simulink model "stpa_brake_manage_maintain"  (R2022a)
settings: Solver=VariableStepAuto  StartTime=0.0  StopTime=10.0  RelTol=1e-3
settings Model: Creator=adije  LastModifiedBy=ayj
settings DebuggingCC: UnconnectedInputMsg=warning  UnconnectedOutputMsg=warning  UnconnectedLineMsg=warning
settings RTWCC: DLArmComputeVersion=19.05

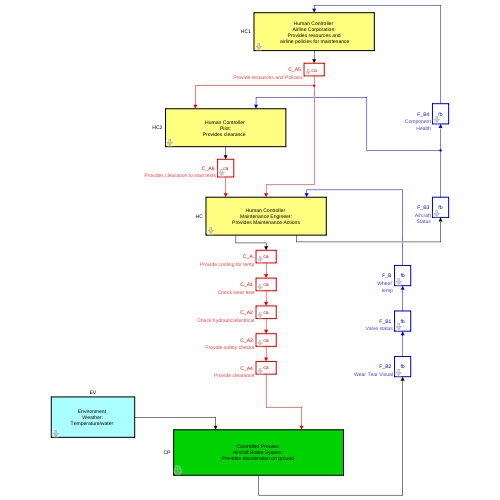
[thumbnail: Simulink's stored preview of the top-level diagram]
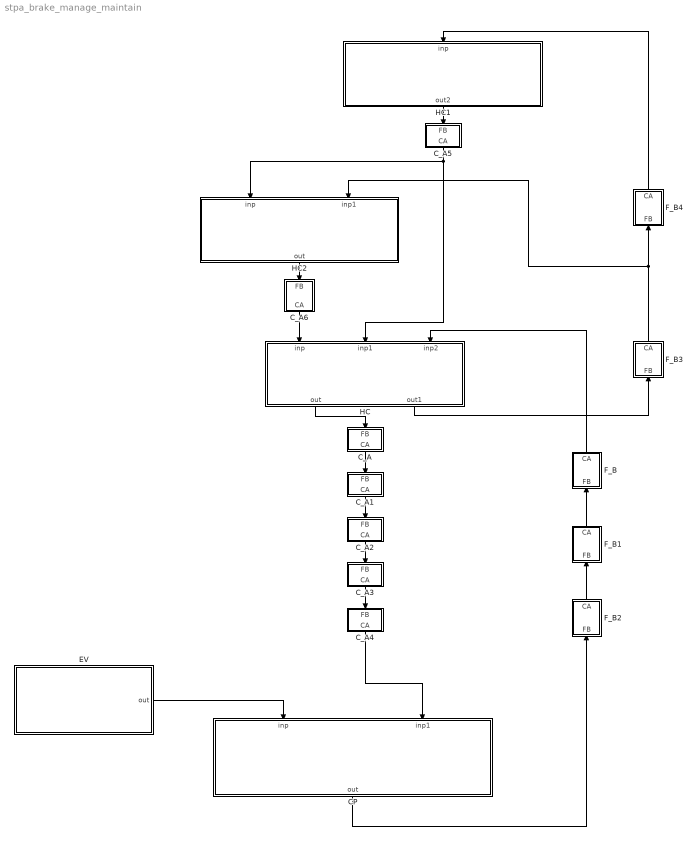
== system stpa_brake_manage_maintain ==
  CP : Subsystem  TreatAsAtomicUnit=on  mask(controlled_process){NAMEFORBLOCK=Aircraft Brake System, DES=Provides deceleration on ground}
      mask prompts: NAMEFORBLOCK "Provide a name for Block"; DES "Provide a description of Responsibility"
      mask help: Say what this controlled process does
      settings: RTWFcnNameOpts=Use subsystem name  RTWFileNameOpts=Use function name
      mask DialogControl Control2 Prompt: ADD Input
      mask DialogControl Control2 Callback:
      | set_param(gcb,'LinkStatus', 'none');
      | h = add_block('simulink/Sources/In1', [gcb '/inp'], 'MakeNameUnique', 'on');
      | hg = add_block('simulink/Sinks/Terminator', [gcb '/term'], 'MakeNameUnique', 'on');
      | hname = get_param(h,'PortHandles');
      | hgname = get_param(hg,'PortHandles');
      | add_line(gcb, hname.Outport(1), hgname.Inport(1));
      mask DialogControl Control3 Prompt: ADD Output
      mask DialogControl Control3 Callback:
      | set_param(gcb,'LinkStatus', 'none');
      | h = add_block('simulink/Sinks/Out1', [gcb '/out'], 'MakeNameUnique', 'on');
      | hg = add_block('simulink/Sources/Ground', [gcb '/gnd'], 'MakeNameUnique', 'on');
      | hname = get_param(h,'PortHandles');
      | hgname = get_param(hg,'PortHandles');
      | add_line(gcb, hgname.Outport(1), hname.Inport(1));
      mask DialogControl Control4 Prompt: REM Input
      mask DialogControl Control4 Callback:
      | set_param(gcb,'LinkStatus', 'none');
      | a=find_system(gcb,'SearchDepth',2,'LookUnderMasks','all','BlockType','Inport');
      | if ~isempty(a)
      | b=get_param(a{1},'PortConnectivity');
      | delete_block(a{1});
      | delete_block(b.DstBlock);
      | delete_line(find_system(gcb, 'SearchDepth',2,'LookUnderMasks','all','FindAll', 'on', 'Type', 'line', 'Connected', 'off'))
      | end
      mask DialogControl Control5 Prompt: REM Output
      mask DialogControl Control5 Callback:
      | set_param(gcb,'LinkStatus', 'none');
      | a=find_system(gcb,'SearchDepth',2,'LookUnderMasks','all','BlockType','Outport');
      | if ~isempty(a)
      | b=get_param(a{1},'PortConnectivity');
      | delete_block(a{1});
      | delete_block(b.SrcBlock);
      | delete_line(find_system(gcb, 'SearchDepth',2,'LookUnderMasks','all','FindAll', 'on', 'Type', 'line', 'Connected', 'off'))
      | end
      mask Display: disp(['Controlled Process \n' NAMEFORBLOCK ':\n' DES])
  C_A : Subsystem  TreatAsAtomicUnit=on  mask(control_action){DES=Provide cooling for temp, UCA1=[#H6] Not providing when temp high, UCA2=[#H6] Providing cooling when not required, UCA3=[#H6] Provide cooling before temprature check, UCA4=[#H6] Provide too long / too short (temp high/low)}
      mask prompts: DES "Provide a description of Control Action"; UCA1 "Not providing causes hazard [link Hazard]"; UCA2 "Providing causes hazard [link Hazard]"; UCA3 "Too early, too late, out of order [link Hazard]"; UCA4 "Stopped too soon, applied too long [link Hazard]"
      mask help:
      | <Source> <Type> <Control Action> <Context> <Link to Hazards>
      | Source = System Above, Type = {provided, not provided ..], Control Action = command
      | from the description, Context = While/When .. Always link to a hazard
      mask init:
      | set_param(gcb,'LinkStatus', 'none');
      settings: AttributesFormatString=%<DES>  RTWFcnNameOpts=Use subsystem name  RTWFileNameOpts=Use function name
      mask Display: disp('ca')
  C_A1 : Subsystem  TreatAsAtomicUnit=on  mask(control_action){DES=Check wear tear, UCA1=[#H7, #H6] Not providing regular checks, UCA2=, UCA3=[#H6] Providing too late, UCA4=[#H7] Takes too long to check}
      mask prompts: DES "Provide a description of Control Action"; UCA1 "Not providing causes hazard [link Hazard]"; UCA2 "Providing causes hazard [link Hazard]"; UCA3 "Too early, too late, out of order [link Hazard]"; UCA4 "Stopped too soon, applied too long [link Hazard]"
      mask help:
      | <Source> <Type> <Control Action> <Context> <Link to Hazards>
      | Source = System Above, Type = {provided, not provided ..], Control Action = command
      | from the description, Context = While/When .. Always link to a hazard
      mask init:
      | set_param(gcb,'LinkStatus', 'none');
      settings: AttributesFormatString=%<DES>  RTWFcnNameOpts=Use subsystem name  RTWFileNameOpts=Use function name
      mask Display: disp('ca')
  C_A2 : Subsystem  TreatAsAtomicUnit=on  mask(control_action){DES=Check hydraulic/electrical, UCA1=[#H6] Not providing before take off, UCA2=, UCA3=[#H6] Too late (hurried work), UCA4=[#H6] Stopping check too soon (assuming)}
      mask prompts: DES "Provide a description of Control Action"; UCA1 "Not providing causes hazard [link Hazard]"; UCA2 "Providing causes hazard [link Hazard]"; UCA3 "Too early, too late, out of order [link Hazard]"; UCA4 "Stopped too soon, applied too long [link Hazard]"
      mask help:
      | <Source> <Type> <Control Action> <Context> <Link to Hazards>
      | Source = System Above, Type = {provided, not provided ..], Control Action = command
      | from the description, Context = While/When .. Always link to a hazard
      mask init:
      | set_param(gcb,'LinkStatus', 'none');
      settings: AttributesFormatString=%<DES>  RTWFcnNameOpts=Use subsystem name  RTWFileNameOpts=Use function name
      mask Display: disp('ca')
  C_A3 : Subsystem  TreatAsAtomicUnit=on  mask(control_action){DES=Provide safety checks, UCA1=[#H5] Not proving safety before tests, UCA2=, UCA3=[#H5] Providing too late (after tests begin), UCA4=[#H5] Providing but not removing safety equipment after checks}
      mask prompts: DES "Provide a description of Control Action"; UCA1 "Not providing causes hazard [link Hazard]"; UCA2 "Providing causes hazard [link Hazard]"; UCA3 "Too early, too late, out of order [link Hazard]"; UCA4 "Stopped too soon, applied too long [link Hazard]"
      mask help:
      | <Source> <Type> <Control Action> <Context> <Link to Hazards>
      | Source = System Above, Type = {provided, not provided ..], Control Action = command
      | from the description, Context = While/When .. Always link to a hazard
      mask init:
      | set_param(gcb,'LinkStatus', 'none');
      settings: AttributesFormatString=%<DES>  RTWFcnNameOpts=Use subsystem name  RTWFileNameOpts=Use function name
      mask Display: disp('ca')
  C_A4 : Subsystem  TreatAsAtomicUnit=on  mask(control_action){DES=Provide clearance, UCA1=[#H7], UCA2=, UCA3=[#H7, #H6] providing improper clearance, UCA4=}
      mask prompts: DES "Provide a description of Control Action"; UCA1 "Not providing causes hazard [link Hazard]"; UCA2 "Providing causes hazard [link Hazard]"; UCA3 "Too early, too late, out of order [link Hazard]"; UCA4 "Stopped too soon, applied too long [link Hazard]"
      mask help:
      | <Source> <Type> <Control Action> <Context> <Link to Hazards>
      | Source = System Above, Type = {provided, not provided ..], Control Action = command
      | from the description, Context = While/When .. Always link to a hazard
      mask init:
      | set_param(gcb,'LinkStatus', 'none');
      settings: AttributesFormatString=%<DES>  RTWFcnNameOpts=Use subsystem name  RTWFileNameOpts=Use function name
      mask Display: disp('ca')
  C_A5 : Subsystem  TreatAsAtomicUnit=on  mask(control_action){DES=Provide resources and Policies, UCA1=[#H4, #H6] Not providing maintenance resources and replacements, UCA2=[#H6] Provided policies are incorrect, UCA3=[#H6] Period of routine checks large, UCA4=[#H6] No consistent and continuous training/monitoring}
      mask prompts: DES "Provide a description of Control Action"; UCA1 "Not providing causes hazard [link Hazard]"; UCA2 "Providing causes hazard [link Hazard]"; UCA3 "Too early, too late, out of order [link Hazard]"; UCA4 "Stopped too soon, applied too long [link Hazard]"
      mask help:
      | <Source> <Type> <Control Action> <Context> <Link to Hazards>
      | Source = System Above, Type = {provided, not provided ..], Control Action = command
      | from the description, Context = While/When .. Always link to a hazard
      mask init:
      | set_param(gcb,'LinkStatus', 'none');
      settings: AttributesFormatString=%<DES>  RTWFcnNameOpts=Use subsystem name  RTWFileNameOpts=Use function name
      mask Display: disp('ca')
  C_A6 : Subsystem  TreatAsAtomicUnit=on  mask(control_action){DES=Provides clearance to start tests, UCA1=[#H7] not providing clearance even when clear, UCA2=[#H5] Provided clearance when unsafe, UCA3=[#H5] Provided clearance when unsafe, UCA4=}
      mask prompts: DES "Provide a description of Control Action"; UCA1 "Not providing causes hazard [link Hazard]"; UCA2 "Providing causes hazard [link Hazard]"; UCA3 "Too early, too late, out of order [link Hazard]"; UCA4 "Stopped too soon, applied too long [link Hazard]"
      mask help:
      | <Source> <Type> <Control Action> <Context> <Link to Hazards>
      | Source = System Above, Type = {provided, not provided ..], Control Action = command
      | from the description, Context = While/When .. Always link to a hazard
      mask init:
      | set_param(gcb,'LinkStatus', 'none');
      settings: AttributesFormatString=%<DES>  RTWFcnNameOpts=Use subsystem name  RTWFileNameOpts=Use function name
      mask Display: disp('ca')
  EV : Subsystem  TreatAsAtomicUnit=on  mask(environment){NAMEFORBLOCK=Weather, DES=Temperature/water}
      mask prompts: NAMEFORBLOCK "Provide a name for Block"; DES "Provide a description of Interaction"
      mask help: Say how this environment interacts with the system
      mask init:
      | set_param(gcb,'LinkStatus', 'none');
      settings: RTWFcnNameOpts=Use subsystem name  RTWFileNameOpts=Use function name
      mask DialogControl Control2 Prompt: ADD Input
      mask DialogControl Control2 Callback:
      | h = add_block('simulink/Sources/In1', [gcb '/inp'], 'MakeNameUnique', 'on');
      | hg = add_block('simulink/Sinks/Terminator', [gcb '/term'], 'MakeNameUnique', 'on');
      | hname = get_param(h,'PortHandles');
      | hgname = get_param(hg,'PortHandles');
      | add_line(gcb, hname.Outport(1), hgname.Inport(1));
      mask DialogControl Control3 Prompt: ADD Output
      mask DialogControl Control3 Callback:
      | h = add_block('simulink/Sinks/Out1', [gcb '/out'], 'MakeNameUnique', 'on');
      | hg = add_block('simulink/Sources/Ground', [gcb '/gnd'], 'MakeNameUnique', 'on');
      | hname = get_param(h,'PortHandles');
      | hgname = get_param(hg,'PortHandles');
      | add_line(gcb, hgname.Outport(1), hname.Inport(1));
      mask DialogControl Control4 Prompt: REM Input
      mask DialogControl Control4 Callback:
      | a=find_system(gcb,'SearchDepth',2,'LookUnderMasks','all','BlockType','Inport');
      | if ~isempty(a)
      | b=get_param(a{1},'PortConnectivity');
      | delete_block(a{1});
      | delete_block(b.DstBlock);
      | delete_line(find_system(gcb, 'SearchDepth',2,'LookUnderMasks','all','FindAll', 'on', 'Type', 'line', 'Connected', 'off'))
      | end
      mask DialogControl Control5 Prompt: REM Output
      mask DialogControl Control5 Callback:
      | a=find_system(gcb,'SearchDepth',2,'LookUnderMasks','all','BlockType','Outport');
      | if ~isempty(a)
      | b=get_param(a{1},'PortConnectivity');
      | delete_block(a{1});
      | delete_block(b.SrcBlock);
      | delete_line(find_system(gcb, 'SearchDepth',2,'LookUnderMasks','all','FindAll', 'on', 'Type', 'line', 'Connected', 'off'))
      | end
      mask Display: disp(['Environment \n' NAMEFORBLOCK ':\n' DES])
  F_B : Subsystem  TreatAsAtomicUnit=on  mask(feedback){DES=Wheel \n temp}
      mask prompts: DES "Provide a description"
      mask help: Say what this feeds back from the system
      mask init:
      | set_param(gcb,'LinkStatus', 'none');
      settings: AttributesFormatString=%<DES>  RTWFcnNameOpts=Use subsystem name  RTWFileNameOpts=Use function name
      mask Display: disp('fb')
  F_B1 : Subsystem  TreatAsAtomicUnit=on  mask(feedback){DES=Valve status}
      mask prompts: DES "Provide a description"
      mask help: Say what this feeds back from the system
      mask init:
      | set_param(gcb,'LinkStatus', 'none');
      settings: AttributesFormatString=%<DES>  RTWFcnNameOpts=Use subsystem name  RTWFileNameOpts=Use function name
      mask Display: disp('fb')
  F_B2 : Subsystem  TreatAsAtomicUnit=on  mask(feedback){DES=Wear Tear Visual}
      mask prompts: DES "Provide a description"
      mask help: Say what this feeds back from the system
      mask init:
      | set_param(gcb,'LinkStatus', 'none');
      settings: AttributesFormatString=%<DES>  RTWFcnNameOpts=Use subsystem name  RTWFileNameOpts=Use function name
      mask Display: disp('fb')
  F_B3 : Subsystem  TreatAsAtomicUnit=on  mask(feedback){DES=Aircraft\n Status}
      mask prompts: DES "Provide a description"
      mask help: Say what this feeds back from the system
      mask init:
      | set_param(gcb,'LinkStatus', 'none');
      settings: AttributesFormatString=%<DES>  RTWFcnNameOpts=Use subsystem name  RTWFileNameOpts=Use function name
      mask Display: disp('fb')
  F_B4 : Subsystem  TreatAsAtomicUnit=on  mask(feedback){DES=Component\n Health}
      mask prompts: DES "Provide a description"
      mask help: Say what this feeds back from the system
      mask init:
      | set_param(gcb,'LinkStatus', 'none');
      settings: AttributesFormatString=%<DES>  RTWFcnNameOpts=Use subsystem name  RTWFileNameOpts=Use function name
      mask Display: disp('fb')
  HC : Subsystem  TreatAsAtomicUnit=on  mask(human_controller){NAMEFORBLOCK=Maintenance Engineer, DES=Provides Maintenance Actions}
      mask prompts: NAMEFORBLOCK "Provide a name for Block"; DES "Provide a description of Responsibility"
      mask help: Say what this human controller does
      mask init:
      | set_param(gcb,'LinkStatus','none')
      settings: RTWFcnNameOpts=Use subsystem name  RTWFileNameOpts=Use function name
      mask DialogControl Control2 Prompt: ADD Input
      mask DialogControl Control2 Callback:
      | h = add_block('simulink/Sources/In1', [gcb '/inp'], 'MakeNameUnique', 'on');
      | hg = add_block('simulink/Sinks/Terminator', [gcb '/term'], 'MakeNameUnique', 'on');
      | hname = get_param(h,'PortHandles');
      | hgname = get_param(hg,'PortHandles');
      | add_line(gcb, hname.Outport(1), hgname.Inport(1));
      mask DialogControl Control3 Prompt: ADD Output
      mask DialogControl Control3 Callback:
      | h = add_block('simulink/Sinks/Out1', [gcb '/out'], 'MakeNameUnique', 'on');
      | hg = add_block('simulink/Sources/Ground', [gcb '/gnd'], 'MakeNameUnique', 'on');
      | hname = get_param(h,'PortHandles');
      | hgname = get_param(hg,'PortHandles');
      | add_line(gcb, hgname.Outport(1), hname.Inport(1));
      mask DialogControl Control4 Prompt: REM Input
      mask DialogControl Control4 Callback:
      | a=find_system(gcb,'SearchDepth',2,'LookUnderMasks','all','BlockType','Inport');
      | if ~isempty(a)
      | b=get_param(a{1},'PortConnectivity');
      | delete_block(a{1});
      | delete_block(b.DstBlock);
      | delete_line(find_system(gcb, 'SearchDepth',2,'LookUnderMasks','all','FindAll', 'on', 'Type', 'line', 'Connected', 'off'))
      | end
      mask DialogControl Control5 Prompt: REM Output
      mask DialogControl Control5 Callback:
      | a=find_system(gcb,'SearchDepth',2,'LookUnderMasks','all','BlockType','Outport');
      | if ~isempty(a)
      | b=get_param(a{1},'PortConnectivity');
      | delete_block(a{1});
      | delete_block(b.SrcBlock);
      | delete_line(find_system(gcb, 'SearchDepth',2,'LookUnderMasks','all','FindAll', 'on', 'Type', 'line', 'Connected', 'off'))
      | end
      mask Display: disp(['Human Controller \n' NAMEFORBLOCK ':\n' DES])
  HC1 : Subsystem  TreatAsAtomicUnit=on  mask(human_controller){NAMEFORBLOCK=Airline Corporation, DES=Provides resources and\n airline policies for maintenance}
      mask prompts: NAMEFORBLOCK "Provide a name for Block"; DES "Provide a description of Responsibility"
      mask help: Say what this human controller does
      mask init:
      | set_param(gcb,'LinkStatus','none')
      settings: RTWFcnNameOpts=Use subsystem name  RTWFileNameOpts=Use function name
      mask DialogControl Control2 Prompt: ADD Input
      mask DialogControl Control2 Callback:
      | h = add_block('simulink/Sources/In1', [gcb '/inp'], 'MakeNameUnique', 'on');
      | hg = add_block('simulink/Sinks/Terminator', [gcb '/term'], 'MakeNameUnique', 'on');
      | hname = get_param(h,'PortHandles');
      | hgname = get_param(hg,'PortHandles');
      | add_line(gcb, hname.Outport(1), hgname.Inport(1));
      mask DialogControl Control3 Prompt: ADD Output
      mask DialogControl Control3 Callback:
      | h = add_block('simulink/Sinks/Out1', [gcb '/out'], 'MakeNameUnique', 'on');
      | hg = add_block('simulink/Sources/Ground', [gcb '/gnd'], 'MakeNameUnique', 'on');
      | hname = get_param(h,'PortHandles');
      | hgname = get_param(hg,'PortHandles');
      | add_line(gcb, hgname.Outport(1), hname.Inport(1));
      mask DialogControl Control4 Prompt: REM Input
      mask DialogControl Control4 Callback:
      | a=find_system(gcb,'SearchDepth',2,'LookUnderMasks','all','BlockType','Inport');
      | if ~isempty(a)
      | b=get_param(a{1},'PortConnectivity');
      | delete_block(a{1});
      | delete_block(b.DstBlock);
      | delete_line(find_system(gcb, 'SearchDepth',2,'LookUnderMasks','all','FindAll', 'on', 'Type', 'line', 'Connected', 'off'))
      | end
      mask DialogControl Control5 Prompt: REM Output
      mask DialogControl Control5 Callback:
      | a=find_system(gcb,'SearchDepth',2,'LookUnderMasks','all','BlockType','Outport');
      | if ~isempty(a)
      | b=get_param(a{1},'PortConnectivity');
      | delete_block(a{1});
      | delete_block(b.SrcBlock);
      | delete_line(find_system(gcb, 'SearchDepth',2,'LookUnderMasks','all','FindAll', 'on', 'Type', 'line', 'Connected', 'off'))
      | end
      mask Display: disp(['Human Controller \n' NAMEFORBLOCK ':\n' DES])
  HC2 : Subsystem  TreatAsAtomicUnit=on  mask(human_controller){NAMEFORBLOCK=Pilot, DES=Provides clearance}
      mask prompts: NAMEFORBLOCK "Provide a name for Block"; DES "Provide a description of Responsibility"
      mask help: Say what this human controller does
      mask init:
      | set_param(gcb,'LinkStatus','none')
      settings: RTWFcnNameOpts=Use subsystem name  RTWFileNameOpts=Use function name
      mask DialogControl Control2 Prompt: ADD Input
      mask DialogControl Control2 Callback:
      | h = add_block('simulink/Sources/In1', [gcb '/inp'], 'MakeNameUnique', 'on');
      | hg = add_block('simulink/Sinks/Terminator', [gcb '/term'], 'MakeNameUnique', 'on');
      | hname = get_param(h,'PortHandles');
      | hgname = get_param(hg,'PortHandles');
      | add_line(gcb, hname.Outport(1), hgname.Inport(1));
      mask DialogControl Control3 Prompt: ADD Output
      mask DialogControl Control3 Callback:
      | h = add_block('simulink/Sinks/Out1', [gcb '/out'], 'MakeNameUnique', 'on');
      | hg = add_block('simulink/Sources/Ground', [gcb '/gnd'], 'MakeNameUnique', 'on');
      | hname = get_param(h,'PortHandles');
      | hgname = get_param(hg,'PortHandles');
      | add_line(gcb, hgname.Outport(1), hname.Inport(1));
      mask DialogControl Control4 Prompt: REM Input
      mask DialogControl Control4 Callback:
      | a=find_system(gcb,'SearchDepth',2,'LookUnderMasks','all','BlockType','Inport');
      | if ~isempty(a)
      | b=get_param(a{1},'PortConnectivity');
      | delete_block(a{1});
      | delete_block(b.DstBlock);
      | delete_line(find_system(gcb, 'SearchDepth',2,'LookUnderMasks','all','FindAll', 'on', 'Type', 'line', 'Connected', 'off'))
      | end
      mask DialogControl Control5 Prompt: REM Output
      mask DialogControl Control5 Callback:
      | a=find_system(gcb,'SearchDepth',2,'LookUnderMasks','all','BlockType','Outport');
      | if ~isempty(a)
      | b=get_param(a{1},'PortConnectivity');
      | delete_block(a{1});
      | delete_block(b.SrcBlock);
      | delete_line(find_system(gcb, 'SearchDepth',2,'LookUnderMasks','all','FindAll', 'on', 'Type', 'line', 'Connected', 'off'))
      | end
      mask Display: disp(['Human Controller \n' NAMEFORBLOCK ':\n' DES])
  wires:
  HC/1(out) -> C_A/1(FB)
  C_A/1(CA) -> C_A1/1(FB)
  F_B/1(CA) -> HC/3(inp2)
  C_A1/1(CA) -> C_A2/1(FB)
  C_A2/1(CA) -> C_A3/1(FB)
  C_A3/1(CA) -> C_A4/1(FB)
  C_A4/1(CA) -> CP/2(inp1)
  EV/1(out) -> CP/1(inp)
  F_B1/1(CA) -> F_B/1(FB)
  F_B2/1(CA) -> F_B1/1(FB)
  HC/2(out1) -> F_B3/1(FB)
  F_B3/1(CA) -> HC2/2(inp1), F_B4/1(FB)
  C_A5/1(CA) -> HC2/1(inp), HC/2(inp1)
  CP/1(out) -> F_B2/1(FB)
  HC2/1(out) -> C_A6/1(FB)
  C_A6/1(CA) -> HC/1(inp)
  F_B4/1(CA) -> HC1/1(inp)
  HC1/1(out2) -> C_A5/1(FB)

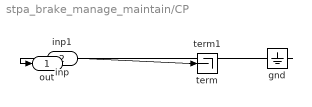
== system stpa_brake_manage_maintain/CP ==
  inp : Inport
  inp1 : Inport  Port=2
  gnd : Ground
  term : Terminator
  term1 : Terminator
  out : Outport
  wires:
  inp/1 -> term/1
  gnd/1 -> out/1
  inp1/1 -> term1/1

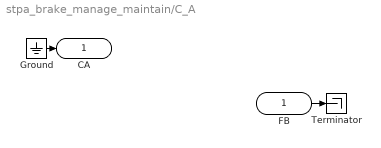
== system stpa_brake_manage_maintain/C_A ==
  FB : Inport
      mask Display:
      | plot([0 60-10],[0 0]);
      | plot([0 0],[0 16]);
      | plot([0 60-10],[16 16]);
      | plot([60-10 60],[16 8]);
      | plot([60-10 60],[0 8]);
  Ground : Ground
  Terminator : Terminator
  CA : Outport
      mask Display:
      | plot([10 65],[0 0]);
      | plot([65-1 65-1],[0 16]);
      | plot([10 65],[16 16]);
      | plot([0 10],[8 16]);
      | plot([0 10],[8 0]);
  wires:
  FB/1 -> Terminator/1
  Ground/1 -> CA/1

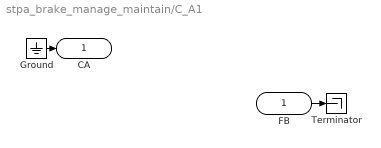
== system stpa_brake_manage_maintain/C_A1 ==
  FB : Inport
      mask Display:
      | plot([0 60-10],[0 0]);
      | plot([0 0],[0 16]);
      | plot([0 60-10],[16 16]);
      | plot([60-10 60],[16 8]);
      | plot([60-10 60],[0 8]);
  Ground : Ground
  Terminator : Terminator
  CA : Outport
      mask Display:
      | plot([10 65],[0 0]);
      | plot([65-1 65-1],[0 16]);
      | plot([10 65],[16 16]);
      | plot([0 10],[8 16]);
      | plot([0 10],[8 0]);
  wires:
  Ground/1 -> CA/1
  FB/1 -> Terminator/1

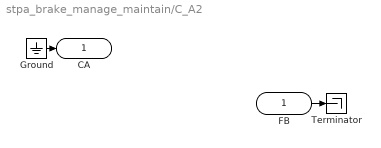
== system stpa_brake_manage_maintain/C_A2 ==
  FB : Inport
      mask Display:
      | plot([0 60-10],[0 0]);
      | plot([0 0],[0 16]);
      | plot([0 60-10],[16 16]);
      | plot([60-10 60],[16 8]);
      | plot([60-10 60],[0 8]);
  Ground : Ground
  Terminator : Terminator
  CA : Outport
      mask Display:
      | plot([10 65],[0 0]);
      | plot([65-1 65-1],[0 16]);
      | plot([10 65],[16 16]);
      | plot([0 10],[8 16]);
      | plot([0 10],[8 0]);
  wires:
  FB/1 -> Terminator/1
  Ground/1 -> CA/1

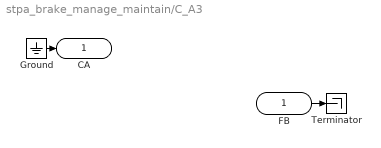
== system stpa_brake_manage_maintain/C_A3 ==
  FB : Inport
      mask Display:
      | plot([0 60-10],[0 0]);
      | plot([0 0],[0 16]);
      | plot([0 60-10],[16 16]);
      | plot([60-10 60],[16 8]);
      | plot([60-10 60],[0 8]);
  Ground : Ground
  Terminator : Terminator
  CA : Outport
      mask Display:
      | plot([10 65],[0 0]);
      | plot([65-1 65-1],[0 16]);
      | plot([10 65],[16 16]);
      | plot([0 10],[8 16]);
      | plot([0 10],[8 0]);
  wires:
  Ground/1 -> CA/1
  FB/1 -> Terminator/1

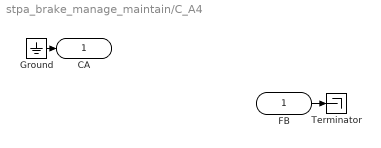
== system stpa_brake_manage_maintain/C_A4 ==
  FB : Inport
      mask Display:
      | plot([0 60-10],[0 0]);
      | plot([0 0],[0 16]);
      | plot([0 60-10],[16 16]);
      | plot([60-10 60],[16 8]);
      | plot([60-10 60],[0 8]);
  Ground : Ground
  Terminator : Terminator
  CA : Outport
      mask Display:
      | plot([10 65],[0 0]);
      | plot([65-1 65-1],[0 16]);
      | plot([10 65],[16 16]);
      | plot([0 10],[8 16]);
      | plot([0 10],[8 0]);
  wires:
  FB/1 -> Terminator/1
  Ground/1 -> CA/1

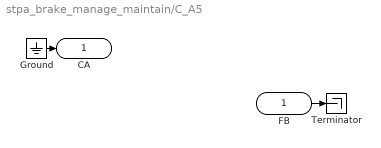
== system stpa_brake_manage_maintain/C_A5 ==
  FB : Inport
      mask Display:
      | plot([0 60-10],[0 0]);
      | plot([0 0],[0 16]);
      | plot([0 60-10],[16 16]);
      | plot([60-10 60],[16 8]);
      | plot([60-10 60],[0 8]);
  Ground : Ground
  Terminator : Terminator
  CA : Outport
      mask Display:
      | plot([10 65],[0 0]);
      | plot([65-1 65-1],[0 16]);
      | plot([10 65],[16 16]);
      | plot([0 10],[8 16]);
      | plot([0 10],[8 0]);
  wires:
  Ground/1 -> CA/1
  FB/1 -> Terminator/1

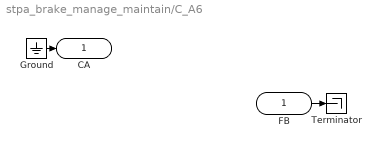
== system stpa_brake_manage_maintain/C_A6 ==
  FB : Inport
      mask Display:
      | plot([0 60-10],[0 0]);
      | plot([0 0],[0 16]);
      | plot([0 60-10],[16 16]);
      | plot([60-10 60],[16 8]);
      | plot([60-10 60],[0 8]);
  Ground : Ground
  Terminator : Terminator
  CA : Outport
      mask Display:
      | plot([10 65],[0 0]);
      | plot([65-1 65-1],[0 16]);
      | plot([10 65],[16 16]);
      | plot([0 10],[8 16]);
      | plot([0 10],[8 0]);
  wires:
  FB/1 -> Terminator/1
  Ground/1 -> CA/1

== system stpa_brake_manage_maintain/EV ==
  gnd : Ground
  out : Outport
  wires:
  gnd/1 -> out/1

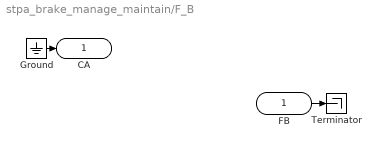
== system stpa_brake_manage_maintain/F_B ==
  FB : Inport
      mask Display:
      | plot([0 60-10],[0 0]);
      | plot([0 0],[0 16]);
      | plot([0 60-10],[16 16]);
      | plot([60-10 60],[16 8]);
      | plot([60-10 60],[0 8]);
  Ground : Ground
  Terminator : Terminator
  CA : Outport
      mask Display:
      | plot([10 65],[0 0]);
      | plot([65-1 65-1],[0 16]);
      | plot([10 65],[16 16]);
      | plot([0 10],[8 16]);
      | plot([0 10],[8 0]);
  wires:
  Ground/1 -> CA/1
  FB/1 -> Terminator/1

== system stpa_brake_manage_maintain/F_B1 ==
  FB : Inport
      mask Display:
      | plot([0 60-10],[0 0]);
      | plot([0 0],[0 16]);
      | plot([0 60-10],[16 16]);
      | plot([60-10 60],[16 8]);
      | plot([60-10 60],[0 8]);
  Ground : Ground
  Terminator : Terminator
  CA : Outport
      mask Display:
      | plot([10 65],[0 0]);
      | plot([65-1 65-1],[0 16]);
      | plot([10 65],[16 16]);
      | plot([0 10],[8 16]);
      | plot([0 10],[8 0]);
  wires:
  FB/1 -> Terminator/1
  Ground/1 -> CA/1

== system stpa_brake_manage_maintain/F_B2 ==
  FB : Inport
      mask Display:
      | plot([0 60-10],[0 0]);
      | plot([0 0],[0 16]);
      | plot([0 60-10],[16 16]);
      | plot([60-10 60],[16 8]);
      | plot([60-10 60],[0 8]);
  Ground : Ground
  Terminator : Terminator
  CA : Outport
      mask Display:
      | plot([10 65],[0 0]);
      | plot([65-1 65-1],[0 16]);
      | plot([10 65],[16 16]);
      | plot([0 10],[8 16]);
      | plot([0 10],[8 0]);
  wires:
  Ground/1 -> CA/1
  FB/1 -> Terminator/1

== system stpa_brake_manage_maintain/F_B3 ==
  FB : Inport
      mask Display:
      | plot([0 60-10],[0 0]);
      | plot([0 0],[0 16]);
      | plot([0 60-10],[16 16]);
      | plot([60-10 60],[16 8]);
      | plot([60-10 60],[0 8]);
  Ground : Ground
  Terminator : Terminator
  CA : Outport
      mask Display:
      | plot([10 65],[0 0]);
      | plot([65-1 65-1],[0 16]);
      | plot([10 65],[16 16]);
      | plot([0 10],[8 16]);
      | plot([0 10],[8 0]);
  wires:
  FB/1 -> Terminator/1
  Ground/1 -> CA/1

== system stpa_brake_manage_maintain/F_B4 ==
  FB : Inport
      mask Display:
      | plot([0 60-10],[0 0]);
      | plot([0 0],[0 16]);
      | plot([0 60-10],[16 16]);
      | plot([60-10 60],[16 8]);
      | plot([60-10 60],[0 8]);
  Ground : Ground
  Terminator : Terminator
  CA : Outport
      mask Display:
      | plot([10 65],[0 0]);
      | plot([65-1 65-1],[0 16]);
      | plot([10 65],[16 16]);
      | plot([0 10],[8 16]);
      | plot([0 10],[8 0]);
  wires:
  Ground/1 -> CA/1
  FB/1 -> Terminator/1

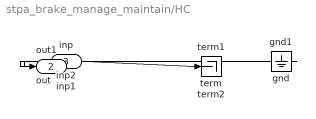
== system stpa_brake_manage_maintain/HC ==
  inp : Inport
  inp1 : Inport  Port=2
  inp2 : Inport  Port=3
  gnd : Ground
  gnd1 : Ground
  term : Terminator
  term1 : Terminator
  term2 : Terminator
  out : Outport
  out1 : Outport  Port=2
  wires:
  inp/1 -> term/1
  gnd/1 -> out/1
  inp1/1 -> term1/1
  gnd1/1 -> out1/1
  inp2/1 -> term2/1

== system stpa_brake_manage_maintain/HC1 ==
  inp : Inport
  gnd2 : Ground
  term : Terminator
  out2 : Outport
  wires:
  gnd2/1 -> out2/1
  inp/1 -> term/1

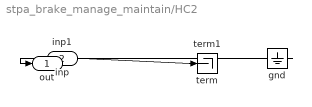
== system stpa_brake_manage_maintain/HC2 ==
  inp : Inport
  inp1 : Inport  Port=2
  gnd : Ground
  term : Terminator
  term1 : Terminator
  out : Outport
  wires:
  inp/1 -> term/1
  gnd/1 -> out/1
  inp1/1 -> term1/1
